simulink model "SOC_Estimation_Coulomb_Counting"  (R2024b)
settings: Solver=VariableStepAuto  StartTime=0.0  StopTime=3600*5  RelTol=1e-3
undefined symbols (not defined in the file): Ion, Lithium
libraries: spsBatteryLib x1, spsCurrentMeasurementLib x1, spsDCMachineLib x1, sps_lib x1
settings Model: Creator=yeswa  LastModifiedBy=yeswa

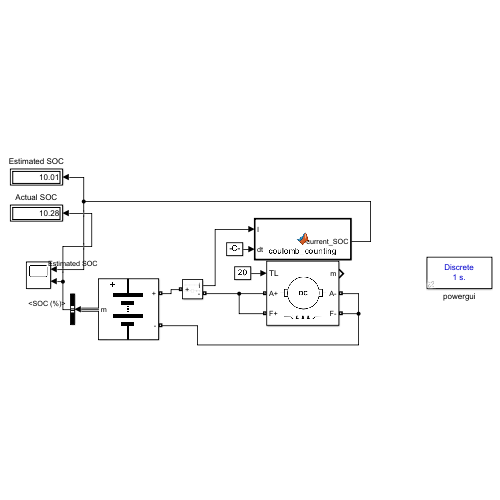
[thumbnail: Simulink's stored preview of the top-level diagram]
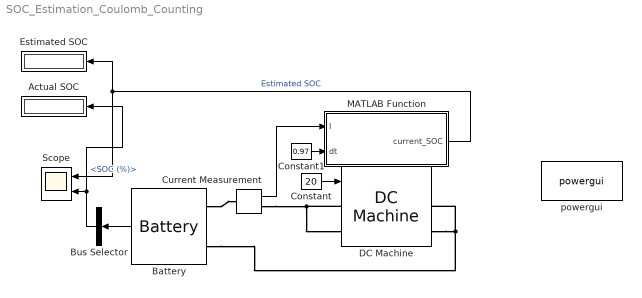
== system SOC_Estimation_Coulomb_Counting ==
  Actual SOC : Display
  Battery : spsBatteryLib/Battery  BatType=Lithium-Ion  NomV=12  NomQ=500  SOC=100  Batt_Tr=30  PresetModel=on  MaxQ=500  MinV=9  FullV=13.9678  Dis_rate=217.3913  R=0.00024  Normal_OP=452.1739  expZone="[12.9646      24.5652]"
  Bus Selector : BusSelector  OutputSignals=SOC (%)
  Constant : Constant  Value=20
  Constant1 : Constant  Value=0.97
  Current Measurement : spsCurrentMeasurementLib/Current Measurement  PhasorSimulation=off  OutputType=Complex  PSBequivalent=0
  DC Machine : spsDCMachineLib/DC Machine  PresetModel=01: 5HP 240V 1750RPM Field:300V  MechanicalLoad=Torque TL  FieldType=Wound  ShowDetailedParameters=on  MeasurementBus=off  RLa=[2.581 0.028]  RLf=[281.2 156]  Laf=0.9483  MachineConstant=Torque constant (N.m/A)  Ke=1.8  Kt=1.8  J=0.02215  Bm=0.002953  Tf=0.5161  w0=1  Ifinit=0  TsPowergui=0  TsBlock=-1
  Estimated SOC : Display
  MATLAB Function : MATLAB Function  TreatAsAtomicUnit=on
  Scope : Scope  NumInputPorts=2
  powergui : sps_lib/powergui  Priority=1  SimulationMode=Discrete  SampleTime=1  frequency=60  Iterations=50  frequencyindice=0  Pbase=100e6  ErrMax=1e-4  UnitsV=kV  UnitsW=MW  buscounter=0  FunctionMessages=off  echomessages=off  EnableUseOfTLC=off  CurrentSourceSwitches=off  DisableSnubberDevices=off  DisableRonSwitches=off  DisableVfSwitches=off  DisplayEquations=off  AutomaticDiscreteSolvers=off  SolverType=Tustin/Backward Euler (TBE)  Interpol=off  ExternalGateDelay=off  methode=off  Ts=100  x0status=blocks  SPID=on  SwTol=0  HookPort=off  NonlinearTolerance=1e-4  nMaxIteration=100  ContinueOnMaxIteration=off  RestoreLinks=warning  ResistiveCurrentMeasurement=off  Frange=[0:2:500]  Ylog=off  Xlog=on  ShowGrid=off  save=off  variable=ZData  structure=0  ZoomFFT=off  StartTime=0.0  cycles=1  DisplayStyle=1  fundamental=60  FreqAxis=off  MaxFrequency=1000  frequencyindicesteady=1  RmsSteady=1  display=off
  wires:
  Battery/1 -> Bus Selector/1
  Bus Selector/1 -> Scope/2, Actual SOC/1  "<SOC (%)>"
  Constant/1 -> DC Machine/1
  Constant1/1 -> MATLAB Function/2(dt)
  Current Measurement/1 -> MATLAB Function/1(I)
  MATLAB Function/1(current_SOC) -> Scope/1, Estimated SOC/1  "Estimated SOC"
  connections:
  DC Machine/LConn1 -- Current Measurement/RConn1 -- DC Machine/LConn2
  Battery/LConn2 -- DC Machine/RConn2 -- DC Machine/RConn1
  Battery/LConn1 -- Current Measurement/LConn1

== matlab function SOC_Estimation_Coulomb_Counting/MATLAB Function ==
  settings: updateMethod=DISCRETE
  data: I input; current_SOC output; dt input
function current_SOC = coulomb_counting(I, dt)
    persistent SOC
    persistent C_bat
    persistent step

    if isempty(SOC)
        SOC = 100;           % Initial SOC [%]
        C_bat = 500 * 3600;  % Battery capacity [As]
        step = 0;            % initialize step counter
    end

    % Increment step count
    step = step + 1;

    % Update SOC (discharge: I > 0 reduces SOC)
    dSOC = -(I * dt) / C_bat * 100;
    SOC = SOC + dSOC;

    % Limit SOC between 0–100
    SOC = max(0, min(100, SOC));

    % Print debug info for first 500 steps
    if step <= 500
        fprintf('Step: %d | Current: %.2f A | dSOC: %.6f %% | SOC: %.4f %%\n', ...
                int32(step), I, dSOC, SOC);
    end

    % Return current SOC
    current_SOC = SOC;
end
